simulink model "foc_sensorless_am13x"  (R2025b)
settings: Solver=FixedStepAuto  StartTime=0.0  StopTime=10  RelTol=1e-3  EnableMultiTasking=on
PostLoadFcn:
  | foc_sensorless_am13x_data;
values from neighbouring files (symbols this model uses):
  inverter = mcb.getInverterParameters('BoostXL-DRV8305')    [foc_sensorless_am13x_data.m]
  PI_params = mcb.getPIControllerParameters(pmsm, inverter, PU_System, T_pwm, Ts, Ts_speed)    [foc_sensorless_am13x_data.m]
  pmsm = mcb.getPMSMParameters('Teknic2310P')    [foc_sensorless_am13x_data.m]
  PU_System = mcb.getPUSystemParameters(pmsm, inverter)    [foc_sensorless_am13x_data.m]
  RAMP_STEP_SIZE = Id_init_assumed / N_ramp_steps    (= 0.00025)    [foc_sensorless_am13x_data.m]
  Speed_openLoop_RPM = Speed_openLoop_PU*pmsm.N_base    [foc_sensorless_am13x_data.m]
  T_pwm = 1 / PWM_frequency    (= 5e-05)    [foc_sensorless_am13x_data.m]
  Tclosedloop_stepTime = 5    [foc_sensorless_am13x_data.m]
  Ts = T_pwm    (= 5e-05)    [foc_sensorless_am13x_data.m]
  Ts_motor = T_pwm / 2    (= 2.5e-05)    [foc_sensorless_am13x_data.m]
  Ts_speed = 10 * Ts    (= 0.0005)    [foc_sensorless_am13x_data.m]
  Tspeedchange_stepTime = 7    [foc_sensorless_am13x_data.m]
undefined symbols (not defined in the file or in its folder): ADC_0_INST, DL_ADC_clearInterruptStatus, DL_ADC_INT_NUMBER1, DL_MCPWM_disableTBCLK, target
libraries: mcbcontrolslib x11, mcbeeMathTransformLib x5, simulink x5, slpidlib x3, peripheral_library_blocks_am13x x2, mcbhdlcontrolslib x2, mcbsensorlessestimatorlib x2, mcbpositiondecoderlib x2, mcbplantlib x1, autolibpmsmexterior x1, simulink_extras x1
(part 1 of 2)
settings Model: Creator=a1255762  LastModifiedBy=a1255762
settings SolverCC: AutoInsertRateTranBlk=on
settings OptimizationCC: DefaultParameterBehavior=Inlined  GainParamInheritBuiltInType=on  UseFloatMulNetSlope=on  DefaultUnderspecifiedDataType=single  UseSpecifiedMinMax=on  InlineInvariantSignals=on  StrengthReduction=on  PassReuseOutputArgsAs=Individual arguments  ZeroExternalMemoryAtStartup=off  ZeroInternalMemoryAtStartup=off  NoFixptDivByZeroProtection=on  EfficientFloat2IntCast=on  MaxStackSize=64  OptimizeBlockOrder=speed  OptimizationPriority=Speed  OptimizationCustomize=off  MultiThreadedLoops=on  AutoScheduleForLoops=on  EfficientTunableParamExpr=on
settings DebuggingCC: MultiTaskDSMMsg=none  ParameterPrecisionLossMsg=none  ParameterTunabilityLossMsg=error
settings HardwareCC: ProdBitPerPointer=32.0  ProdBitPerSizeT=32.0  ProdBitPerPtrDiffT=32.0  ProdLargestAtomicInteger=Long  ProdLargestAtomicFloat=Double  ProdWordSize=32.0  ProdLongLongMode=on  ProdHWDeviceType=ARM Compatible->ARM Cortex
settings ModelReferenceCC: ModelReferenceNumInstancesAllowed=Single
settings SFSimCC: MATLABDynamicMemAlloc=off
settings RTWCC: SystemTargetFile=ert.tlc  HardwareBoard=AM13E230x  TemplateMakefile=ert_default_tmf  Toolchain=TI ARM Clang Compiler AM13x | gmake  BuildConfiguration=Faster Runs  Description=Embedded Coder
settings CodeAppCC: ForceParamTrailComments=on  IgnoreCustomStorageClasses=off  MaxIdLength=256.0  OperatorAnnotations=on  SimulinkDataObjDesc=on  SFDataObjDesc=on  InsertBlockDesc=on
settings ERTTargetCC: ExtModeTransport=3.0  ExtModeStaticAlloc=on  ExtModeMexFile=ext_xcp  ExtModeIntrfLevel=Level2 - Open  ERTCustomFileTemplate=AM13x_codertarget_file_process.tlc  CodeReplacementLibrary=AM13x_TMU  CombineSignalStateStructs=on  SuppressErrorStatus=on  SupportAbsoluteTime=off  SubcomponentCodeInterfacePackaging=Nonreusable function  SupportNonFinite=off  SupportComplex=off

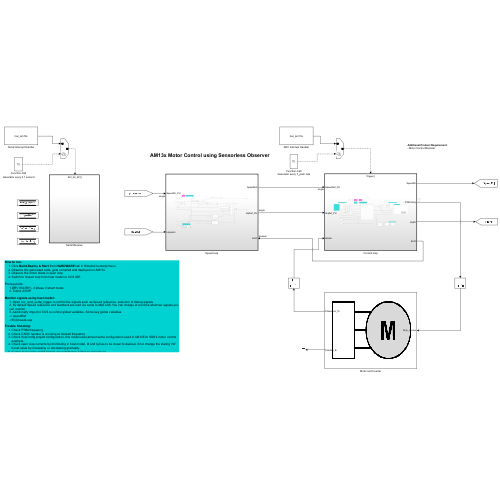
[thumbnail: Simulink's stored preview of the top-level diagram]
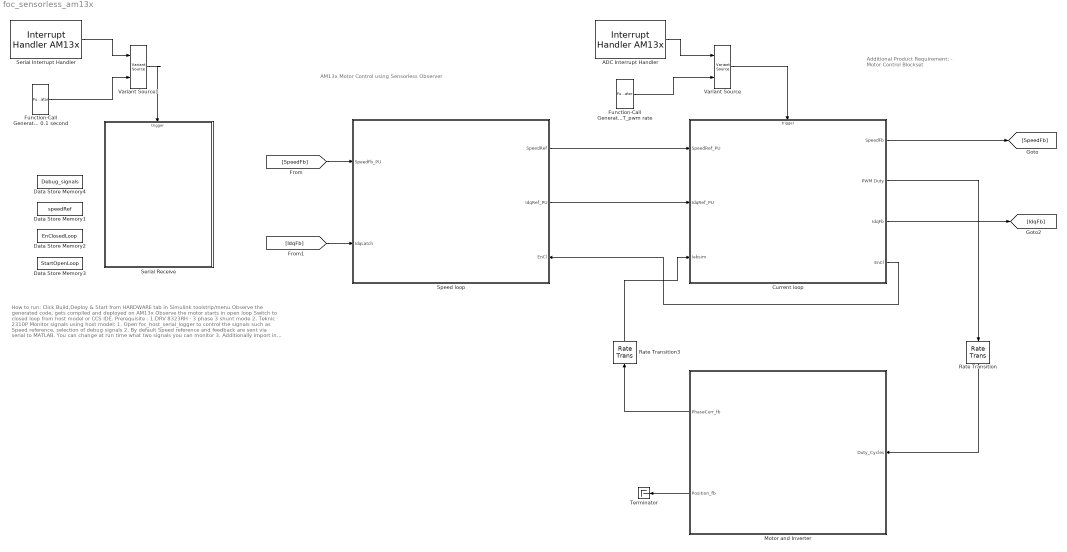
== system foc_sensorless_am13x ==
  note: Additional Product Requirement:
      | - Motor Control Blockset
  note: AM13x Motor Control using Sensorless Observer
  note: How to run:
      | Click Build,Deploy & Start from HARDWARE tab in Simulink toolstrip/menu
      | Observe the generated code, gets compiled and deployed on AM13x
      | Observe the motor starts in open loop
      | Switch to closed loop from host model or CCS IDE.
      |
      | Prerequisite :
      | 1.DRV 8323RH - 3 phase 3 shunt mode
      | 2. Teknic 2310P
      |
      | Monitor signals using host model:
      | 1. Open foc_host_serial_logger to control the signals such as Speed reference, selection of debug signals
      | 2. By default Speed reference and feedback are sent via serial to MATLAB. You can change at run time what two signals you can monitor
      | 3. Additionally import in CCS to control global variables. Some key global variables
      | -> speedRef
      | ->EnClosedLoop
      |
      | Trouble Shooting:
      | Check PWM frequency
      | Check if ADC handler is occuring at desired frequency
      | Check SysConfig project configuration, this model uses almost same configuration used in AM13E2x SDK's motor control example.
      | Check open loop currents by monitoring in host model. Id and Iq has to be closer to desired, if not change the staring Vd/boost value by increasing or decreasing gradually.
      | If open loop works and if signals are satisfactory switch to closed loop
  ADC Interrupt Handler : peripheral_library_blocks_am13x/Interrupt Handler AM13x  InterruptHandler=MTR1_FOC_INT1_Handler  PrologHandler=DL_ADC_clearInterruptStatus(ADC_0_INST, DL_ADC_INT_NUMBER1)
      settings: SourceProductName=Embedded Coder Support Package for AM13X - Peripheral Blocks
  Current loop : Subsystem
  Data Store Memory1 : DataStoreMemory  DataStoreName=speedRef  InitialValue=0.2*pmsm.N_base  ShowAdditionalParam=off  OutDataTypeStr=single
  Data Store Memory2 : DataStoreMemory  DataStoreName=EnClosedLoop  ShowAdditionalParam=off  OutDataTypeStr=boolean
  Data Store Memory3 : DataStoreMemory  DataStoreName=StartOpenLoop  ShowAdditionalParam=off  OutDataTypeStr=boolean
  Data Store Memory4 : DataStoreMemory  DataStoreName=Debug_signals  InitialValue=1  ShowAdditionalParam=off  OutDataTypeStr=uint16
  Function-Call Generator every 0.1 second : FunctionCallGenerator  SampleTime=.1
  Function-Call Generator every T_pwm rate : FunctionCallGenerator  SampleTime=T_pwm
  Motor and Inverter : Subsystem
      mask Display: image('mcb_pmsmfoc_motor.png');
  Rate Transition : RateTransition  Deterministic=off  OutPortSampleTime=Ts/2
  Rate Transition3 : RateTransition  Deterministic=off
  Serial Interrupt Handler : peripheral_library_blocks_am13x/Interrupt Handler AM13x  InterruptHandler=MW_SERIAL_RX_UC_IRQ_HANDLER  PrologHandler=Uart_Hal_InterruptHandler(&mw_am13x_serial_UartInstance)
      settings: SourceProductName=Embedded Coder Support Package for AM13X - Peripheral Blocks
  Serial Receive : Subsystem  SystemSampleTime=1e-3
  Speed loop : Subsystem  TreatAsAtomicUnit=on  SystemSampleTime=Ts_speed
      settings: PortSchema="{\"entries\":[{\"content\":{\"sides\":[{\"content\":{\"connectorIds\":[\"In1\",\"In2\"]},\"type\":\"ConnectorPlacement.EquallySpacedRectSide\",\"uuid\":\"b506ce2e-5969-464b-b6d0-26d5d9421673\"},{\"content\":{\"connectorIds\":[\"Out1\",\"Out2\",\"In3\"],\"side\":\"RIGHT\"},\"type\":\"ConnectorPlacement.EquallySpacedRectSide\",\"uuid\":\"4d96be12-936e-4168-b358-ef77535e2717\"},{\"content\":{\"side\":\"TOP\"},\"type\":\"ConnectorPlacement.EquallySpacedRectSide\",\"uuid\":\"e3c638c2-3aa9-4a35-855d-e235e847103f\"}]},\"type\":\"ConnectorPlacement.EquallySpacedConnector\",\"uuid\":\"420ee1be-7685-485e-b81d-67f311436300\"}],\"packageUris\":[\"http://schema.mathworks.com/mf0/Connector/R2020b\"],\"version\":\"1.0\"}"
  Terminator : Terminator
  Variant Source : VariantSource  VariantControlMode=sim codegen switching  OutputFunctionCall=on  VariantControls={(codegen), (sim)}
  Variant Source1 : VariantSource  VariantControlMode=sim codegen switching  OutputFunctionCall=on  VariantControls={(codegen), (sim)}
  wires:
  Rate Transition/1 -> Motor and Inverter/1(Duty_Cycles)
  Current loop/1(SpeedFb) -> [SpeedFb]
  Current loop/2(PWM Duty) -> Rate Transition/1
  Current loop/3(IdqFb) -> [IdqFb]
  ADC Interrupt Handler/1 -> Variant Source/1
  Function-Call Generator every T_pwm rate/1 -> Variant Source/2
  Variant Source/1 -> Current loop/Trigger
  Motor and Inverter/1(PhaseCurr_fb) -> Rate Transition3/1
  Rate Transition3/1 -> Current loop/3(Iabsim)
  [SpeedFb] -> Speed loop/1(SpeedFb_PU)
  [IdqFb] -> Speed loop/2(IdqLatch)
  Motor and Inverter/2(Position_fb) -> Terminator/1
  Speed loop/1(SpeedRef) -> Current loop/1(SpeedRef_PU)
  Speed loop/2(IdqRef_PU) -> Current loop/2(IdqRef_PU)
  Current loop/4(EnCl) -> Speed loop/3(EnCl)
  Function-Call Generator every 0.1 second/1 -> Variant Source1/2
  Serial Interrupt Handler/1 -> Variant Source1/1
  Variant Source1/1 -> Serial Receive/Trigger

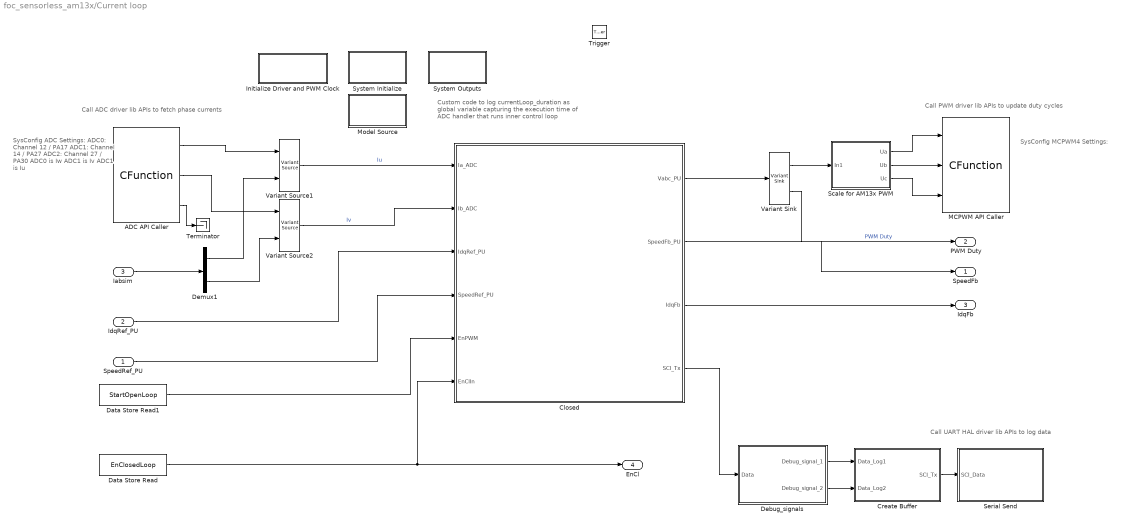
== system foc_sensorless_am13x/Current loop ==
  note: SysConfig ADC Settings:
      |
      | ADC0: Channel 12 / PA17
      | ADC1: Channel 14 / PA27
      | ADC2: Channel 27 / PA30
      |
      |
      | ADC0 is Iw
      | ADC1 is Iv
      | ADC1 is Iu
  note: Custom code to log currentLoop_duration as global variable capturing the execution time of ADC handler that runs inner control loop
  note: Call ADC driver lib APIs to fetch phase currents
  note: Call PWM driver lib APIs to update duty cycles
  note: Call UART HAL driver lib APIs to log data
  note: SysConfig MCPWM4 Settings:
  SpeedRef_PU : Inport  OutDataTypeStr=single
  IdqRef_PU : Inport  Port=2
  Iabsim : Inport  Port=3
  Trigger : TriggerPort  TriggerType=function-call  VariantControl=(inherit)  PortDimensions=1
  " ADC API Caller" : CFunction  CodeGenUsesSimCustomCode=off  CodegenOutputCode=|  CustomHeaderFile=|
      CodegenOutputCode=|
      | /* Read ADC conversion results from respective result registers */ 
      | Iw = DL_ADC_readResult(ADC_0_RESULT_INST, DL_ADC_SOC_NUMBER0);
      | Iv = DL_ADC_readResult(ADC_1_RESULT_INST, DL_ADC_SOC_NUMBER0);
      | Iu = DL_ADC_readResult(ADC_2_RESULT_INST, DL_ADC_SOC_NUMBER0);
      CustomHeaderFile=|
      | dl_adc.h
      | hw_memmap.h
      | ti_sdk_dl_config.h
  "Closed " : Subsystem  RTWFcnName=MTR1_FOC_INT1_Handler
      settings: RTWFcnNameOpts=User specified
  Create Buffer : Subsystem
  Data Store Read : DataStoreRead  DataStoreName=EnClosedLoop  IndexOptions=Index vector (dialog)  Indices=1  OutputSizes=1
  Data Store Read1 : DataStoreRead  DataStoreName=StartOpenLoop  IndexOptions=Index vector (dialog)  Indices=1  OutputSizes=1
  Debug_signals : Subsystem
  Demux1 : Demux  Outputs=2
  Initialize Driver and PWM Clock : Subsystem  TreatAsAtomicUnit=on
  MCPWM API Caller : CFunction  CodeGenUsesSimCustomCode=off  CodegenOutputCode=|  CustomHeaderFile=|
      CodegenOutputCode=|
      | DL_MCPWM_setCounterCompareShadowValue(MTR1_MCPWM_BASE_INST, DL_MCPWM_COUNTER_COMPARE_1A, Ua);
      | DL_MCPWM_setCounterCompareShadowValue(MTR1_MCPWM_BASE_INST, DL_MCPWM_COUNTER_COMPARE_1B, Ua);
      | DL_MCPWM_setCounterCompareShadowValue(MTR1_MCPWM_BASE_INST, DL_MCPWM_COUNTER_COMPARE_2A, Ub);
      | DL_MCPWM_setCounterCompareShadowValue(MTR1_MCPWM_BASE_INST, DL_MCPWM_COUNTER_COMPARE_2B, Ub);
      | DL_MCPWM_setCounterCompareShadowValue(MTR1_MCPWM_BASE_INST, DL_MCPWM_COUNTER_COMPARE_3A, Uc);
      | DL_MCPWM_setCounterCompareShadowValue(MTR1_MCPWM_BASE_INST, DL_MCPWM_COUNTER_COMPARE_3B, Uc);
      CustomHeaderFile=|
      | dl_mcpwm.h
      | hw_memmap.h
      | ti_sdk_dl_config.h
  Model Source : Subsystem  mask(Model Source){ShowInLibBrowser=0}
      mask prompts: ShowInLibBrowser "Simulink:masks:CustCodeMaskParam1_MP"
      settings: CopyFcn=cccopyfcn(gcb)  OpenFcn=ccopenfcn('Model Source')
      mask Help: eval('feval(''rtwprivate'',''rtwhelpview'',''rtw_model_source_block'')');
      mask Display: disp('Model\nSource');
  Scale for AM13x PWM : Subsystem
  Serial Send : Subsystem
  System Initialize : Subsystem  mask(System Initialize){ShowInLibBrowser=0}
      mask prompts: ShowInLibBrowser "Simulink:masks:CustCodeMaskParam1_MP"
      settings: CopyFcn=cccopyfcn(gcb)  OpenFcn=ccopenfcn('System Initialize Function')
      mask Help: eval('feval(''rtwprivate'',''rtwhelpview'',''rtw_sys_initialize_block'')');
      mask Display: disp('System\nInitialize');
  System Outputs : Subsystem  mask(System Outputs){ShowInLibBrowser=0}
      mask prompts: ShowInLibBrowser "Simulink:masks:CustCodeMaskParam1_MP"
      settings: CopyFcn=cccopyfcn(gcb)  OpenFcn=ccopenfcn('System Outputs Function')
      mask Help: eval('feval(''rtwprivate'',''rtwhelpview'',''rtw_sys_outputs_block'')');
      mask Display: disp('System\nOutputs');
  Terminator : Terminator
  Variant Sink : VariantSink  VariantControlMode=sim codegen switching  VariantControls={(codegen), (sim)}
  Variant Source1 : VariantSource  VariantControlMode=sim codegen switching  VariantControls={(codegen), (sim)}
  Variant Source2 : VariantSource  VariantControlMode=sim codegen switching  VariantControls={(codegen), (sim)}
  SpeedFb : Outport
  PWM Duty : Outport  Port=2
  IdqFb : Outport  Port=3
  EnCl : Outport  Port=4
  wires:
  " ADC API Caller"/1 -> Variant Source1/1
  Demux1/1 -> Variant Source1/2
  Variant Sink/2 -> PWM Duty/1  "PWM Duty"
  " ADC API Caller"/2 -> Variant Source2/1
  Variant Source1/1 -> "Closed "/1(Ia_ADC)  "Iu"
  Variant Source2/1 -> "Closed "/2(Ib_ADC)  "Iv"
  "Closed "/1(Vabc_PU) -> Variant Sink/1
  "Closed "/2(SpeedFb_PU) -> SpeedFb/1
  "Closed "/3(IdqFb) -> IdqFb/1
  IdqRef_PU/1 -> "Closed "/3(IdqRef_PU)
  SpeedRef_PU/1 -> "Closed "/4(SpeedRef_PU)
  Data Store Read/1 -> EnCl/1, "Closed "/6(EnClIn)
  Demux1/2 -> Variant Source2/2
  Iabsim/1 -> Demux1/1
  Create Buffer/1(SCI_Tx) -> Serial Send/1(SCI_Data)
  "Closed "/4(SCI_Tx) -> Debug_signals/1(Data)
  Debug_signals/2(Debug_signal_2) -> Create Buffer/2(Data_Log2)
  Debug_signals/1(Debug_signal_1) -> Create Buffer/1(Data_Log1)
  " ADC API Caller"/3 -> Terminator/1
  Variant Sink/1 -> Scale for AM13x PWM/1(In1)
  Scale for AM13x PWM/1(Ua) -> MCPWM API Caller/1
  Scale for AM13x PWM/2(Ub) -> MCPWM API Caller/2
  Scale for AM13x PWM/3(Uc) -> MCPWM API Caller/3
  Data Store Read1/1 -> "Closed "/5(EnPWM)

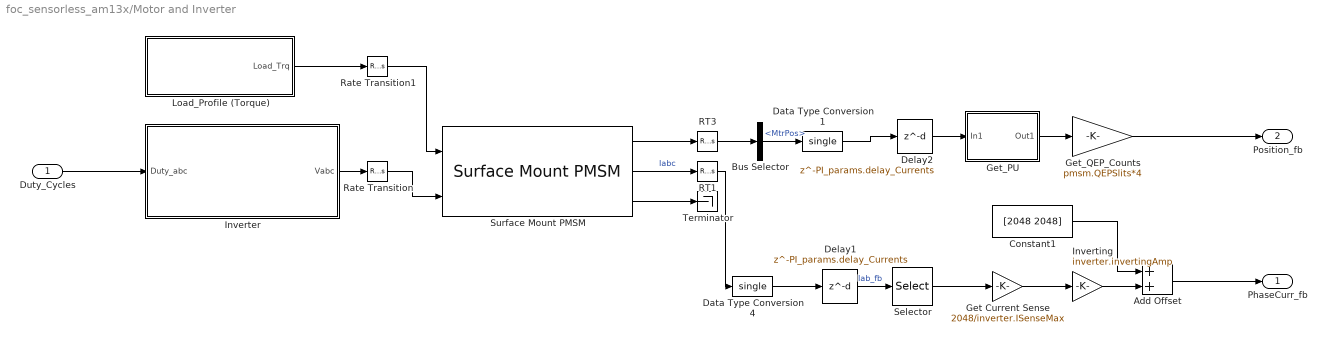
== system foc_sensorless_am13x/Motor and Inverter ==
  Duty_Cycles : Inport
  Add Offset : Sum  OutDataTypeStr=Inherit: Same as first input
  Bus Selector : BusSelector  OutputSignals=MtrPos
  Constant1 : Constant  Value=[2048 2048]  OutDataTypeStr=uint16
  Data Type Conversion1 : DataTypeConversion  OutDataTypeStr=single  RndMeth=Simplest  SaturateOnIntegerOverflow=off
  Data Type Conversion4 : DataTypeConversion  OutDataTypeStr=single  RndMeth=Simplest  SaturateOnIntegerOverflow=off
  Delay1 : Delay  DelayLength=PI_params.delay_Currents
  Delay2 : Delay  DelayLength=PI_params.delay_Currents
  "Get Current Sense " : Gain  Gain=2048/inverter.ISenseMax  OutDataTypeStr=int16  RndMeth=Simplest
  Get_PU : Subsystem
  Get_QEP_Counts : Gain  Gain=pmsm.QEPSlits*4  OutDataTypeStr=uint16  RndMeth=Simplest
  Inverter : Subsystem
  Inverting : Gain  Gain=inverter.invertingAmp  OutDataTypeStr=int16  RndMeth=Simplest
  Load_Profile (Torque) : Subsystem
  RT1 : RateTransition  Deterministic=off  OutPortSampleTime=Ts_motor
  RT3 : RateTransition  Deterministic=off  OutPortSampleTime=Ts_motor
  Rate Transition : RateTransition  Deterministic=off  OutPortSampleTime=Ts_motor
  Rate Transition1 : RateTransition  Deterministic=off  OutPortSampleTime=Ts_motor
  Selector : Selector  InputPortWidth=3  IndexOptions=Index vector (dialog)  Indices=[1 2]  OutputSizes=1
  Surface Mount PMSM : autolibpmsmexterior/Surface Mount PMSM  port_config=Torque  sim_type=Discrete  Ts=Ts_motor  P=pmsm.p  Rs=pmsm.Rs  Ldq_=pmsm.Ld  KConstText=Back-emf constant (Ke):  lambda_pm=pmsm.FluxPM  Ke=pmsm.Ke  Kt=1.323  mechanical=[pmsm.J, pmsm.B, 0]  idq0=[0 0]  theta_init=0  omega_init=0  KConst=pmsm.FluxPM  lambda_pm_calc=0.0096483  RefBlkName='autolibpmsmexterior/Surface Mount PMSM'  aMode=5  Ldq="[0.0002      0.0002]"
  Terminator : Terminator
  PhaseCurr_fb : Outport
  Position_fb : Outport  Port=2
  wires:
  Data Type Conversion1/1 -> Delay2/1
  Bus Selector/1 -> Data Type Conversion1/1  "<MtrPos>"
  Delay1/1 -> Selector/1  "Iab_fb"
  Data Type Conversion4/1 -> Delay1/1
  Duty_Cycles/1 -> Inverter/1(Duty_abc)
  RT3/1 -> Bus Selector/1
  Rate Transition1/1 -> Surface Mount PMSM/1
  Surface Mount PMSM/3 -> Terminator/1
  Surface Mount PMSM/2 -> RT1/1  "Iabc"
  Inverter/1(Vabc) -> Rate Transition/1
  Load_Profile (Torque)/1(Load_Trq) -> Rate Transition1/1
  Rate Transition/1 -> Surface Mount PMSM/2
  Surface Mount PMSM/1 -> RT3/1
  RT1/1 -> Data Type Conversion4/1
  Get_QEP_Counts/1 -> Position_fb/1
  "Get Current Sense "/1 -> Inverting/1
  Constant1/1 -> Add Offset/1
  Delay2/1 -> Get_PU/1(In1)
  Get_PU/1(Out1) -> Get_QEP_Counts/1
  Add Offset/1 -> PhaseCurr_fb/1
  Selector/1 -> "Get Current Sense "/1
  Inverting/1 -> Add Offset/2

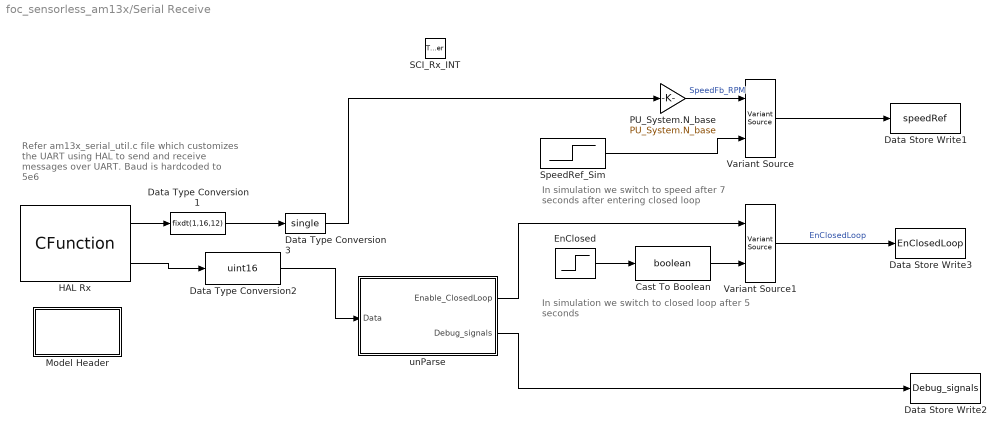
== system foc_sensorless_am13x/Serial Receive ==
  note: Refer am13x_serial_util.c file which customizes the UART using HAL to send and receive messages over UART. Baud is hardcoded to 5e6
  note: In simulation we switch to speed after 7 seconds after entering closed loop
  note: In simulation we switch to closed loop after 5 seconds
  SCI_Rx_INT : TriggerPort  TriggerType=function-call  VariantControl=Variant
  Cast To Boolean : DataTypeConversion  OutDataTypeStr=boolean  SaturateOnIntegerOverflow=off  RndMeth=Floor
  Data Store Write1 : DataStoreWrite  DataStoreName=speedRef  IndexOptions=Index vector (dialog)  Indices=1  OutputSizes=1
  Data Store Write2 : DataStoreWrite  DataStoreName=Debug_signals  IndexOptions=Index vector (dialog)  Indices=1  OutputSizes=1
  Data Store Write3 : DataStoreWrite  DataStoreName=EnClosedLoop  IndexOptions=Index vector (dialog)  Indices=1  OutputSizes=1
  Data Type Conversion1 : DataTypeConversion  OutDataTypeStr=fixdt(1,16,12)  ConvertRealWorld=Stored Integer (SI)  RndMeth=Simplest  SaturateOnIntegerOverflow=off
  Data Type Conversion2 : DataTypeConversion  OutDataTypeStr=uint16  RndMeth=Simplest  SaturateOnIntegerOverflow=off
  Data Type Conversion3 : DataTypeConversion  OutDataTypeStr=single  RndMeth=Simplest  SaturateOnIntegerOverflow=off
  EnClosed : Step  Time=Tclosedloop_stepTime  OutDataTypeStr=single
  HAL Rx : CFunction  CodeGenUsesSimCustomCode=off  CodegenOutputCode=mw_am13x_serial_GetRxData(&SCI_Rx1, &SCI_Rx2);  CustomHeaderFile=|
      | hw_memmap.h
      | ti_sdk_dl_config.h
      | Uart_Hal.h
  Model Header : Subsystem  mask(Model Header){ShowInLibBrowser=0}
      mask prompts: ShowInLibBrowser "Simulink:masks:CustCodeMaskParam1_MP"
      settings: CopyFcn=cccopyfcn(gcb)  OpenFcn=ccopenfcn('Model Header')
      mask Help: eval('feval(''rtwprivate'',''rtwhelpview'',''rtw_model_header_block'')');
      mask Display: disp('Model\nHeader');
  PU_System.N_base : Gain  Gain=PU_System.N_base
  SpeedRef_Sim : Step  Time=Tspeedchange_stepTime  Before=0.2*pmsm.N_base  After=0.3*pmsm.N_base  OutDataTypeStr=single
  Variant Source : VariantSource  VariantControlMode=sim codegen switching  VariantControls={(codegen), (sim)}
  Variant Source1 : VariantSource  VariantControlMode=sim codegen switching  VariantControls={(codegen), (sim)}
  unParse : Subsystem
  wires:
  Data Type Conversion3/1 -> PU_System.N_base/1
  HAL Rx/1 -> Data Type Conversion1/1
  unParse/2(Debug_signals) -> Data Store Write2/1
  Data Type Conversion2/1 -> unParse/1(Data)
  Data Type Conversion1/1 -> Data Type Conversion3/1
  HAL Rx/2 -> Data Type Conversion2/1
  SpeedRef_Sim/1 -> Variant Source/2
  Variant Source/1 -> Data Store Write1/1
  PU_System.N_base/1 -> Variant Source/1  "SpeedFb_RPM"
  Variant Source1/1 -> Data Store Write3/1  "EnClosedLoop"
  EnClosed/1 -> Cast To Boolean/1
  unParse/1(Enable_ClosedLoop) -> Variant Source1/1
  Cast To Boolean/1 -> Variant Source1/2

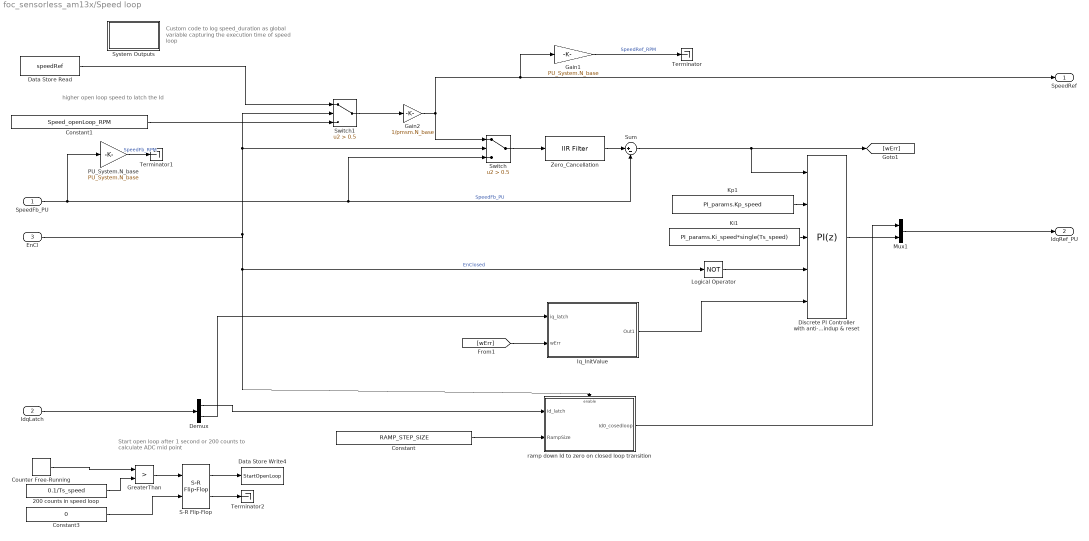
== system foc_sensorless_am13x/Speed loop ==
  note: higher open loop speed to latch the Id
  note: Start open loop after 1 second or 200 counts to calculate ADC mid point
  note: Custom code to log speed_duration as global variable capturing the execution time of speed loop
  SpeedFb_PU : Inport  OutDataTypeStr=single
  IdqLatch : Inport  Port=2
  EnCl : Inport  Port=3  OutDataTypeStr=boolean
  200 counts in speed loop : Constant  Value=0.1/Ts_speed  OutDataTypeStr=uint16
  Constant : Constant  Value=RAMP_STEP_SIZE  OutDataTypeStr=single
  Constant1 : Constant  Value=Speed_openLoop_RPM  OutDataTypeStr=single
  Constant3 : Constant  Value=0  OutDataTypeStr=boolean
  Counter Free-Running : simulink/Sources/Counter Free-Running  NumBits=16  tsamp=-1
  Data Store Read : DataStoreRead  DataStoreName=speedRef  IndexOptions=Index vector (dialog)  Indices=1  OutputSizes=1
  Data Store Write4 : DataStoreWrite  DataStoreName=StartOpenLoop  IndexOptions=Index vector (dialog)  Indices=1  OutputSizes=1
  Demux : Demux  Outputs=2
  Discrete PI Controller with anti-windup & reset : slpidlib/PID Controller  Controller=PI  Form=Parallel  TimeDomain=Discrete-time  UseExternalTs=off  SampleTime=-1  IntegratorMethod=Forward Euler  FilterMethod=Forward Euler  ControllerParametersSource=external  P=1  I=1  UseKiTs=on  D=0  UseExternalDerivativeSource=off  N=100  UseFilter=on  TunerSelectOption=Transfer Function Based (PID Tuner App)  InitialConditionSource=external  InitialConditionForIntegrator=0  InitialConditionForFilter=0  DifferentiatorICPrevScaledInput=0  ExternalReset=level  TrackingMode=off  Kt=1  LimitOutput=on  SatLimitsSource=internal  UpperSaturationLimit=pmsm.I_rated/inverter.ISenseMax  LowerSaturationLimit=-pmsm.I_rated/inverter.ISenseMax  LinearizeAsGain=on  AntiWindupMode=clamping  Kb=1  LimitIntegrator=off  UpperIntegratorSaturationLimit=inf  LowerIntegratorSaturationLimit=-inf  RndMeth=Simplest  POutMin=[]  POutMax=[]  IOutMin=[]  IOutMax=[]  DOutMin=[]  DOutMax=[]  NOutMin=[]  NOutMax=[]  SumOutMin=[]  SumOutMax=[]  SaturationOutDataTypeStr=Inherit: Inherit via back propagation  SaturationOutMin=[]  SaturationOutMax=[]  PParamMin=[]  PParamMax=[]  IParamMin=[]  IParamMax=[]  DParamMin=[]  DParamMax=[]  NParamMin=[]  NParamMax=[]  KbParamMin=[]  KbParamMax=[]  KtParamMin=[]  KtParamMax=[]  KbOutMin=[]  KbOutMax=[]  KtOutMin=[]  KtOutMax=[]  IntegratorOutMin=[]  IntegratorOutMax=[]  FilterOutMin=[]  FilterOutMax=[]  SumI1OutMin=[]  SumI1OutMax=[]  SumI2OutMin=[]  SumI2OutMax=[]  SumI3OutMin=[]  SumI3OutMax=[]  SumI4OutMin=[]  SumI4OutMax=[]  SumDOutMin=[]  SumDOutMax=[]  DifferentiatorOutMin=[]  DifferentiatorOutMax=[]  FilterDiffOutCoefMin=[]  FilterDiffOutCoefMax=[]  ReciprocalOutMin=[]  ReciprocalOutMax=[]  SumDenOutMin=[]  SumDenOutMax=[]  SumNumOutMin=[]  SumNumOutMax=[]  DivideOutMin=[]  DivideOutMax=[]  UdiffTsProdOutMin=[]  UdiffTsProdOutMax=[]  NTsProdOutMin=[]  NTsProdOutMax=[]  UintegralTsProdOutMin=[]  UintegralTsProdOutMax=[]  UngainTsProdOutMin=[]  UngainTsProdOutMax=[]  ClampingZeroOutDataTypeStr=Inherit: Inherit via back propagation  ClampingZeroOutMin=[]  ClampingZeroOutMax=[]  FilterDenConstantOutDataTypeStr=Inherit: Inherit via back propagation  FilterDenConstantOutMin=[]  FilterDenConstantOutMax=[]  PCopyOutDataTypeStr=Inherit: Inherit via back propagation  PCopyOutMin=[]  PCopyOutMax=[]  NCopyOutDataTypeStr=Inherit: Inherit via back propagation  NCopyOutMin=[]  NCopyOutMax=[]  IntegratorContinuousStateAttributes=''  IntegratorStateMustResolveToSignalObject=off  IntegratorRTWStateStorageClass=Auto  FilterContinuousStateAttributes=''  FilterStateMustResolveToSignalObject=off  FilterRTWStateStorageClass=Auto  ParallelPVariant=ExternalParameters  IdealPVariant=Disabled  IVariant=ExternalParameters  DVariant=Disabled  IntegratorVariant=Discrete  SatVariant=Enabled  AWVariant=DiscClampingParallel  PCopyVariant=Disabled  TRVariant=Disabled  FdbkBlocksVariant=Forward  IdealPFdbkVariant=Disabled  SatFdbkVariant=Disabled  DerivativeFilterVariant=Disabled  NVariant=Disabled  NCopyVariant=Disabled_SignalSpec  FilterICVariant=Disabled  IntegratorICVariant=ExternalICs  ExternalResetVariant=ExternalReset  TRSumVariant=Passthrough  SumFdbkVariant=Disabled  SumVariant=Sum_PI  TsampFilterVariant=InternalTs  TsampNgainVariant=Passthrough  TsampIntegralVariant=Disabled_SignalSpec  ExternalSaturationOutDataTypeStr=Inherit: Same as second input  DerivativeSourceVariant=Disabled  PreIntVariant=InternalPreInt
      settings: LibrarySourceBlock=mcbcontrolslib/PI Controller
  Gain1 : Gain  Gain=PU_System.N_base
  Gain2 : Gain  Gain=1/pmsm.N_base
  GreaterThan : RelationalOperator  Operator=>  OutDataTypeStr=boolean  RndMeth=Simplest  InputSameDT=off
  Iq_InitValue : Subsystem
  Ki1 : Constant  Value=PI_params.Ki_speed*single(Ts_speed)  OutDataTypeStr=dataType  SampleTime=-1
  Kp1 : Constant  Value=PI_params.Kp_speed  OutDataTypeStr=dataType  SampleTime=-1
  Logical Operator : Logic  Operator=NOT  IconShape=distinctive  AllPortsSameDT=off  OutDataTypeStr=boolean
  Mux1 : Mux  Inputs=2
  PU_System.N_base : Gain  Gain=PU_System.N_base
  S-R Flip-Flop : simulink_extras/Flip Flops/S-R Flip-Flop  initial_condition=0
  Sum : Sum  Inputs=|+-  OutDataTypeStr=Inherit: Same as first input
  Switch : Switch  Criteria=u2 > Threshold  Threshold=0.5  SaturateOnIntegerOverflow=off  InputSameDT=off
  Switch1 : Switch  Criteria=u2 > Threshold  Threshold=0.5  SaturateOnIntegerOverflow=off  InputSameDT=off
  System Outputs : Subsystem  mask(System Outputs){ShowInLibBrowser=0}
      mask prompts: ShowInLibBrowser "Simulink:masks:CustCodeMaskParam1_MP"
      settings: CopyFcn=cccopyfcn(gcb)  OpenFcn=ccopenfcn('System Outputs Function')
      mask Help: eval('feval(''rtwprivate'',''rtwhelpview'',''rtw_sys_outputs_block'')');
      mask Display: disp('System\nOutputs');
  Terminator : Terminator
  Terminator1 : Terminator
  Terminator2 : Terminator
  Zero_Cancellation : mcbcontrolslib/IIR Filter  VariantControl=Low Pass Filter  VariantSelect=Low-pass  FilterConstantInputType=Specify via dialog  Filter_constant=0.01*(Ts_speed/Ts)  InitialOutput=Specify via dialog  InitialOutputValue=0  ExternalReset=none  advancedSettings=off  Ts=50e-6  cutOff_freq=353.6777
  ramp down Id to zero on closed loop transition : Subsystem
  SpeedRef : Outport
  IdqRef_PU : Outport  Port=2  OutDataTypeStr=single  VectorParamsAs1DForOutWhenUnconnected=off
  wires:
  Mux1/1 -> IdqRef_PU/1
  Kp1/1 -> Discrete PI Controller with anti-windup & reset/2
  PU_System.N_base/1 -> Terminator1/1  "SpeedFb_RPM"
  Logical Operator/1 -> Discrete PI Controller with anti-windup & reset/4
  Gain1/1 -> Terminator/1  "SpeedRef_RPM"
  SpeedFb_PU/1 -> PU_System.N_base/1, Sum/2, Switch/3  "SpeedFb_PU"
  Discrete PI Controller with anti-windup & reset/1 -> Mux1/2
  Sum/1 -> Discrete PI Controller with anti-windup & reset/1, [wErr]
  Ki1/1 -> Discrete PI Controller with anti-windup & reset/3
  EnCl/1 -> ramp down Id to zero on closed loop transition/Enable, Logical Operator/1, Switch/2, Switch1/2  "EnClosed"
  Switch1/1 -> Gain2/1
  Gain2/1 -> Switch/1, Gain1/1, SpeedRef/1
  Switch/1 -> Zero_Cancellation/1
  IdqLatch/1 -> Demux/1
  Demux/1 -> ramp down Id to zero on closed loop transition/1(Id_latch)
  Constant/1 -> ramp down Id to zero on closed loop transition/2(RampSize)
  Constant1/1 -> Switch1/3
  Demux/2 -> Iq_InitValue/1(iq_latch)
  Iq_InitValue/1(Out1) -> Discrete PI Controller with anti-windup & reset/5
  ramp down Id to zero on closed loop transition/1(Id0_cosedloop) -> Mux1/1
  [wErr] -> Iq_InitValue/2(wErr)
  Data Store Read/1 -> Switch1/1
  Zero_Cancellation/1 -> Sum/1
  S-R Flip-Flop/1 -> Data Store Write4/1
  S-R Flip-Flop/2 -> Terminator2/1
  Counter Free-Running/1 -> GreaterThan/1
  GreaterThan/1 -> S-R Flip-Flop/1
  200 counts in speed loop/1 -> GreaterThan/2
  Constant3/1 -> S-R Flip-Flop/2

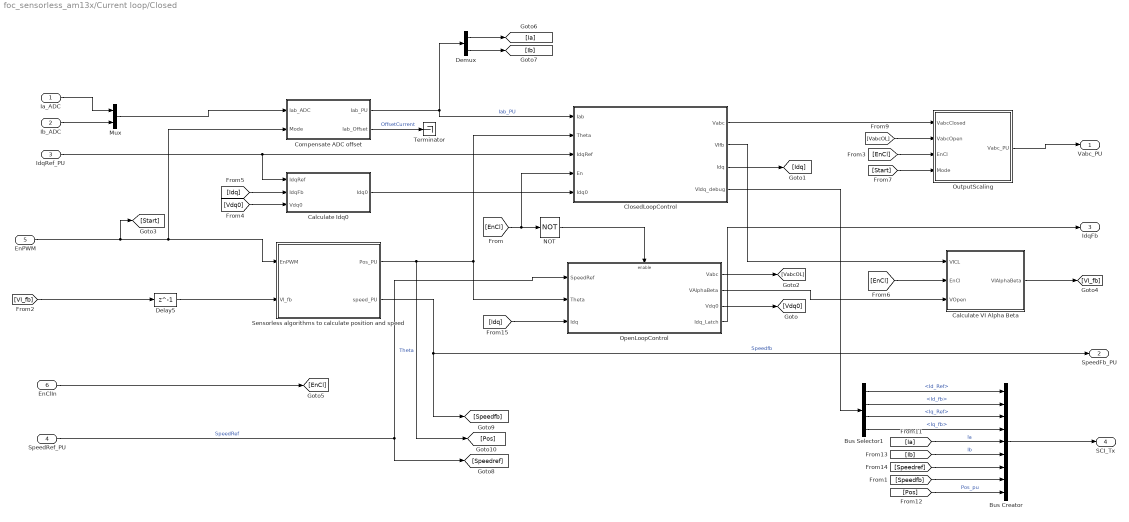
== system foc_sensorless_am13x/Current loop/Closed  ==
  Ia_ADC : Inport
  Ib_ADC : Inport  Port=2
  IdqRef_PU : Inport  Port=3  OutDataTypeStr=dataType  PortDimensions=2
  SpeedRef_PU : Inport  Port=4  OutDataTypeStr=single
  EnPWM : Inport  Port=5
  EnClIn : Inport  Port=6
  Bus Creator : BusCreator  Inputs=9
  Bus Selector1 : BusSelector  OutputSignals=Id_Ref,Id_fb,Iq_Ref,Iq_fb
  Calculate Idq0 : Subsystem
  Calculate VI Alpha Beta : Subsystem
  ClosedLoopControl : Subsystem
  Compensate ADC offset : Subsystem
  Delay5 : Delay  DelayLength=1
  Demux : Demux  Outputs=2
  Mux : Mux  Inputs=2
  NOT : Logic  Operator=NOT  IconShape=distinctive  AllPortsSameDT=off  OutDataTypeStr=boolean
  OpenLoopControl : Subsystem
  OutputScaling : Subsystem
  Sensorless algorithms to calculate position and speed : Subsystem
  Terminator : Terminator
  Vabc_PU : Outport  OutDataTypeStr=single  VectorParamsAs1DForOutWhenUnconnected=off
  SpeedFb_PU : Outport  Port=2
  IdqFb : Outport  Port=3
  SCI_Tx : Outport  Port=4
  wires:
  NOT/1 -> OpenLoopControl/Enable
  OpenLoopControl/2(VAlphaBeta) -> Calculate VI Alpha Beta/3(VOpen)
  [EnCl] -> OutputScaling/3(EnCl)
  Compensate ADC offset/1(Iab_PU) -> Demux/1, ClosedLoopControl/1(Iab)  "Iab_PU"
  [Vdq0] -> Calculate Idq0/3(Vdq0)
  Delay5/1 -> Sensorless algorithms to calculate position and speed/2(VI_fb)
  OpenLoopControl/3(Vdq0) -> [Vdq0]
  Sensorless algorithms to calculate position and speed/1(Pos_PU) -> [Pos], OpenLoopControl/2(Theta), ClosedLoopControl/2(Theta)  "Theta"
  SpeedRef_PU/1 -> [Speedref], OpenLoopControl/1(SpeedRef)  "SpeedRef"
  Calculate Idq0/1(Idq0) -> ClosedLoopControl/5(Idq0)
  [EnCl] -> Calculate VI Alpha Beta/2(EnCl)
  IdqRef_PU/1 -> ClosedLoopControl/3(IdqRef), Calculate Idq0/1(IdqRef)
  [VI_fb] -> Delay5/1
  [VabcOL] -> OutputScaling/2(VabcOpen)
  OutputScaling/1(Vabc_PU) -> Vabc_PU/1
  ClosedLoopControl/3(Idq) -> [Idq]
  [EnCl] -> ClosedLoopControl/4(En), NOT/1
  OpenLoopControl/1(Vabc) -> [VabcOL]
  [Idq] -> Calculate Idq0/2(IdqFb)
  EnClIn/1 -> [EnCl]
  Ib_ADC/1 -> Mux/2
  Ia_ADC/1 -> Mux/1
  Sensorless algorithms to calculate position and speed/2(speed_PU) -> [Speedfb], SpeedFb_PU/1  "Speedfb"
  [Speedfb] -> Bus Creator/8
  [Ia] -> Bus Creator/5  "Ia"
  [Speedref] -> Bus Creator/7
  [Ib] -> Bus Creator/6  "Ib"
  [Pos] -> Bus Creator/9  "Pos_pu"
  Bus Creator/1 -> SCI_Tx/1
  Calculate VI Alpha Beta/1(VIAlphaBeta) -> [VI_fb]
  Demux/1 -> [Ia]
  Mux/1 -> Compensate ADC offset/1(Iab_ADC)
  Demux/2 -> [Ib]
  Bus Selector1/1 -> Bus Creator/1  "<Id_Ref>"
  Bus Selector1/2 -> Bus Creator/2  "<Id_fb>"
  Bus Selector1/3 -> Bus Creator/3  "<Iq_Ref>"
  Bus Selector1/4 -> Bus Creator/4  "<Iq_fb>"
  ClosedLoopControl/1(Vabc) -> OutputScaling/1(VabcClosed)
  ClosedLoopControl/2(VIfb) -> Calculate VI Alpha Beta/1(VICL)
  ClosedLoopControl/4(VIdq_debug) -> Bus Selector1/1
  Compensate ADC offset/2(Iab_Offset) -> Terminator/1  "OffsetCurrent"
  [Idq] -> OpenLoopControl/3(Idq)
  OpenLoopControl/4(Idq_Latch) -> IdqFb/1
  [Start] -> OutputScaling/4(Mode)
  EnPWM/1 -> [Start], Compensate ADC offset/2(Mode), Sensorless algorithms to calculate position and speed/1(EnPWM)

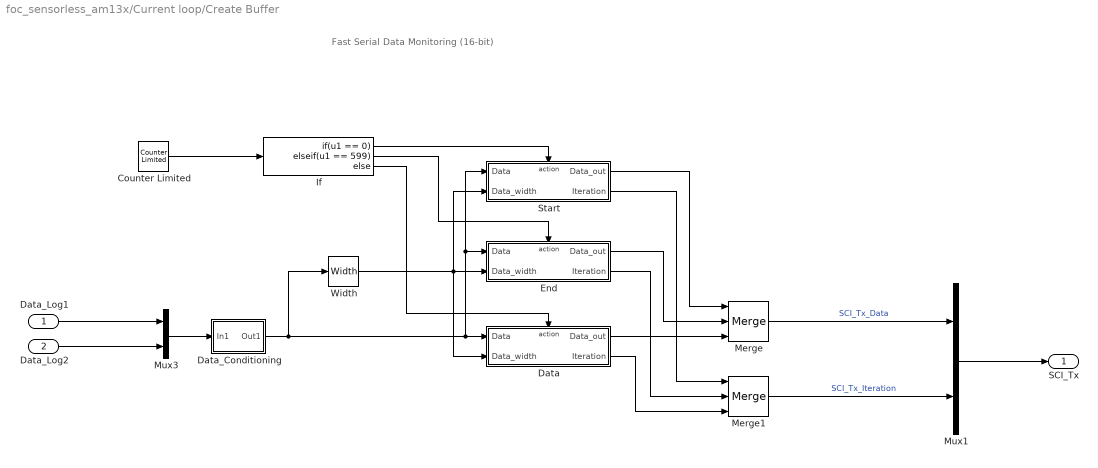
== system foc_sensorless_am13x/Current loop/Create Buffer ==
  note: Fast Serial Data Monitoring (16-bit)
  Data_Log1 : Inport
  Data_Log2 : Inport  Port=2
  Counter Limited : simulink/Sources/Counter Limited  uplimit=599  tsamp=-1
  Data : Subsystem  TreatAsAtomicUnit=on
  Data_Conditioning : Subsystem
  End : Subsystem  TreatAsAtomicUnit=on
  If : If  IfExpression=u1 == 0  ElseIfExpressions=u1 == 599
  Merge : Merge  Inputs=3
  Merge1 : Merge  Inputs=3
  Mux1 : Mux  Inputs=2
  Mux3 : Mux  Inputs=2
  Start : Subsystem  TreatAsAtomicUnit=on
  Width : Width  OutDataTypeMode=All ports same datatype  DataType=uint16
  SCI_Tx : Outport
  wires:
  Data_Conditioning/1(Out1) -> Width/1, Data/1(Data), End/1(Data), Start/1(Data)
  Counter Limited/1 -> If/1
  Data_Log1/1 -> Mux3/1
  Data/1(Data_out) -> Merge/3
  Data_Log2/1 -> Mux3/2
  Width/1 -> Data/2(Data_width), End/2(Data_width), Start/2(Data_width)
  Data/2(Iteration) -> Merge1/3
  End/2(Iteration) -> Merge1/2
  If/1 -> Start/Action
  Start/1(Data_out) -> Merge/1
  Merge1/1 -> Mux1/2  "SCI_Tx_Iteration"
  Mux3/1 -> Data_Conditioning/1(In1)
  Start/2(Iteration) -> Merge1/1
  If/2 -> End/Action
  End/1(Data_out) -> Merge/2
  If/3 -> Data/Action
  Mux1/1 -> SCI_Tx/1
  Merge/1 -> Mux1/1  "SCI_Tx_Data"

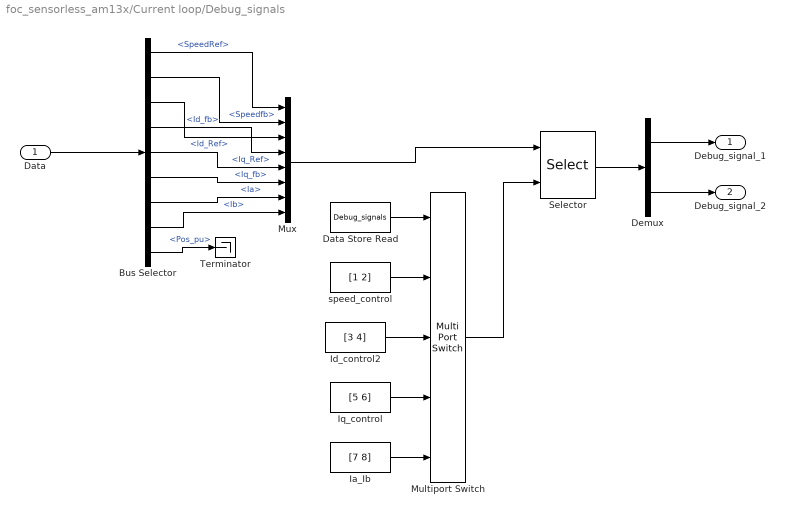
== system foc_sensorless_am13x/Current loop/Debug_signals ==
  Data : Inport
  Bus Selector : BusSelector  OutputSignals=SpeedRef,Speedfb,Id_Ref,Id_fb,Iq_Ref,Iq_fb,Ia,Ib,Pos_pu
  Data Store Read : DataStoreRead  DataStoreName=Debug_signals  IndexOptions=Index vector (dialog)  Indices=1  OutputSizes=1
  Demux : Demux  Outputs=2
  Ia_Ib : Constant  Value=[7 8]  OutDataTypeStr=uint16  SampleTime=-1
  Id_control2 : Constant  Value=[3 4]  OutDataTypeStr=uint16  SampleTime=-1
  Iq_control : Constant  Value=[5 6]  OutDataTypeStr=uint16  SampleTime=-1
  Multiport Switch : MultiPortSwitch  Inputs=4  DiagnosticForDefault=Warning  OutDataTypeStr=uint16  RndMeth=Simplest  SaturateOnIntegerOverflow=off  InputSameDT=off
  Mux : Mux  Inputs=8
  Selector : Selector  InputPortWidth=8  IndexOptions=Index vector (port)  Indices=[1 3]  OutputSizes=1
  Terminator : Terminator
  speed_control : Constant  Value=[1 2]  OutDataTypeStr=uint16  SampleTime=-1
  Debug_signal_1 : Outport
  Debug_signal_2 : Outport  Port=2
  wires:
  Demux/2 -> Debug_signal_2/1
  speed_control/1 -> Multiport Switch/2
  Selector/1 -> Demux/1
  Demux/1 -> Debug_signal_1/1
  Id_control2/1 -> Multiport Switch/3
  Iq_control/1 -> Multiport Switch/4
  Ia_Ib/1 -> Multiport Switch/5
  Multiport Switch/1 -> Selector/2
  Data Store Read/1 -> Multiport Switch/1
  Data/1 -> Bus Selector/1
  Bus Selector/2 -> Mux/2  "<Speedfb>"
  Mux/1 -> Selector/1
  Bus Selector/3 -> Mux/3  "<Id_Ref>"
  Bus Selector/4 -> Mux/4  "<Id_fb>"
  Bus Selector/5 -> Mux/5  "<Iq_Ref>"
  Bus Selector/6 -> Mux/6  "<Iq_fb>"
  Bus Selector/7 -> Mux/7  "<Ia>"
  Bus Selector/8 -> Mux/8  "<Ib>"
  Bus Selector/1 -> Mux/1  "<SpeedRef>"
  Bus Selector/9 -> Terminator/1  "<Pos_pu>"

== system foc_sensorless_am13x/Current loop/Initialize Driver and PWM Clock ==
  C Function : CFunction  CodeGenUsesSimCustomCode=off  CodegenInitializeConditionsCode=|  CodegenTerminateCode=DL_MCPWM_disableTBCLK();  CustomHeaderFile=|
      CodegenInitializeConditionsCode=|
      | /* Power-up adc converter core */
      | DL_ADC_powerUp(ADC_0_INST);
      | DL_ADC_powerUp(ADC_1_INST);
      | DL_ADC_powerUp(ADC_2_INST);
      | DEVICE_DELAY_US(10000); /* 10ms delay*/
      | /* Power-up MCPWM */
      | DL_MCPWM_enableTBCLK();
      | /* uart init */
      | mw_am13x_serial_Init();
      CustomHeaderFile=|
      | dl_gpio.h
      | hw_memmap.h
      | ti_sdk_dl_config.h
      | dl_mcpwm.h
      | dl_adc.h
  Constant1 : Constant  OutDataTypeStr=single
  Event Listener : EventListener  DisableCoverage=on  EventName=reset
  wires:
  Constant1/1 -> C Function/1

== system foc_sensorless_am13x/Current loop/Model Source ==

== system foc_sensorless_am13x/Current loop/Scale for AM13x PWM ==
  note: This gain is to create global variable for these signals, Its a workaround
  In1 : Inport
  Demux : Demux  Outputs=3
  Gain : Gain  OutDataTypeStr=uint16
  Gain1 : Gain  OutDataTypeStr=uint16
  Gain2 : Gain  OutDataTypeStr=uint16
  Scale_to_PWM_Counter_PRD : Gain  Gain=target.PWM_Counter_Period  OutDataTypeStr=uint16  RndMeth=Simplest
  Ua : Outport
  Ub : Outport  Port=2
  Uc : Outport  Port=3
  wires:
  Demux/2 -> Gain1/1
  Gain/1 -> Ua/1  "Ua"
  Demux/3 -> Gain2/1
  Gain2/1 -> Uc/1  "Uc"
  In1/1 -> Scale_to_PWM_Counter_PRD/1
  Demux/1 -> Gain/1
  Scale_to_PWM_Counter_PRD/1 -> Demux/1
  Gain1/1 -> Ub/1  "Ub"

== system foc_sensorless_am13x/Current loop/Serial Send ==
  SCI_Data : Inport
  Demux2 : Demux  Outputs=2
  While Iterator Subsystem : Subsystem  TreatAsAtomicUnit=on
  wires:
  Demux2/2 -> While Iterator Subsystem/2(Iteration)  "SCI_Tx_Iteration"
  Demux2/1 -> While Iterator Subsystem/1(Data)  "SCI_Tx_Data"
  SCI_Data/1 -> Demux2/1

== system foc_sensorless_am13x/Current loop/System Initialize ==

== system foc_sensorless_am13x/Current loop/System Outputs ==

== system foc_sensorless_am13x/Motor and Inverter/Get_PU ==
  In1 : Inport
  Constant : Constant  Value=2*pi  OutDataTypeStr=single
  Gain2 : Gain  Gain=1/(2*pi)  RndMeth=Simplest  OutDataTypeStr=Inherit: Same as input
  Mod : Math  Operator=mod
  Out1 : Outport
  wires:
  Constant/1 -> Mod/2
  In1/1 -> Mod/1
  Mod/1 -> Gain2/1
  Gain2/1 -> Out1/1

== system foc_sensorless_am13x/Motor and Inverter/Inverter ==
  Duty_abc : Inport
  Average-Value Inverter : mcbplantlib/Average-Value Inverter
  Constant2 : Constant  Value=inverter.V_dc  OutDataTypeStr=single  SampleTime=-1
  Data Type Conversion1 : DataTypeConversion  OutDataTypeStr=single  RndMeth=Simplest  SaturateOnIntegerOverflow=off
  Rate Transition3 : RateTransition  Deterministic=off  OutPortSampleTime=Ts_motor
  Vabc : Outport  VectorParamsAs1DForOutWhenUnconnected=off
  wires:
  Average-Value Inverter/1 -> Vabc/1
  Rate Transition3/1 -> Average-Value Inverter/1
  Duty_abc/1 -> Data Type Conversion1/1
  Data Type Conversion1/1 -> Rate Transition3/1
  Constant2/1 -> Average-Value Inverter/2

== system foc_sensorless_am13x/Motor and Inverter/Load_Profile (Torque) ==
  Constant : Constant  Value=.01*pmsm.T_rated  OutDataTypeStr=single  SampleTime=-1
  Data Type Conversion : DataTypeConversion  OutDataTypeStr=single  SaturateOnIntegerOverflow=off  RndMeth=Floor
  IIR Filter : mcbcontrolslib/IIR Filter  VariantControl=Low Pass Filter  VariantSelect=Low-pass  FilterConstantInputType=Specify via dialog  Filter_constant=0.001  InitialOutput=Specify via dialog  InitialOutputValue=0  ExternalReset=none  advancedSettings=off  Ts=50e-6  cutOff_freq=3.1863
  T_load : Step  Time=8  Before=.01*pmsm.T_rated  After=.05*pmsm.T_rated  SampleTime=Ts_motor
  Load_Trq : Outport  VectorParamsAs1DForOutWhenUnconnected=off
  wires:
  IIR Filter/1 -> Load_Trq/1
  Data Type Conversion/1 -> IIR Filter/1
  Constant/1 -> Data Type Conversion/1

== system foc_sensorless_am13x/Serial Receive/Model Header ==

== system foc_sensorless_am13x/Serial Receive/unParse ==
  Data : Inport
  Bitwise Operator : simulink/Logic and Bit Operations/Bitwise Operator  logicop=AND  UseBitMask=on  BitMask=hex2dec('0001')  BitMaskRealWorld=Stored Integer
  Bitwise Operator1 : simulink/Logic and Bit Operations/Bitwise Operator  logicop=AND  UseBitMask=on  BitMask=hex2dec('00F0')  BitMaskRealWorld=Stored Integer
  Data Type Conversion3 : DataTypeConversion  OutDataTypeStr=boolean  RndMeth=Simplest  SaturateOnIntegerOverflow=off
  Data Type Conversion4 : DataTypeConversion  OutDataTypeStr=uint16  RndMeth=Simplest  SaturateOnIntegerOverflow=off
  Shift Arithmetic1 : ArithShift  BitShiftNumber=4
  Enable_ClosedLoop : Outport
  Debug_signals : Outport  Port=2
  wires:
  Data Type Conversion3/1 -> Enable_ClosedLoop/1
  Shift Arithmetic1/1 -> Data Type Conversion4/1
  Data Type Conversion4/1 -> Debug_signals/1
  Bitwise Operator/1 -> Data Type Conversion3/1
  Data/1 -> Bitwise Operator1/1, Bitwise Operator/1
  Bitwise Operator1/1 -> Shift Arithmetic1/1

== system foc_sensorless_am13x/Speed loop/Iq_InitValue ==
  iq_latch : Inport
  wErr : Inport  Port=2
  Add : Sum  Inputs=-+  RndMeth=Simplest  OutDataTypeStr=Inherit: Same as first input
  Kp2 : Constant  Value=PI_params.Kp_speed  OutDataTypeStr=dataType  SampleTime=-1
  Product : Product  RndMeth=Simplest  OutDataTypeStr=Inherit: Same as first input
  Out1 : Outport
  wires:
  wErr/1 -> Product/2
  Add/1 -> Out1/1
  Product/1 -> Add/1
  Kp2/1 -> Product/1
  iq_latch/1 -> Add/2

== system foc_sensorless_am13x/Speed loop/System Outputs ==

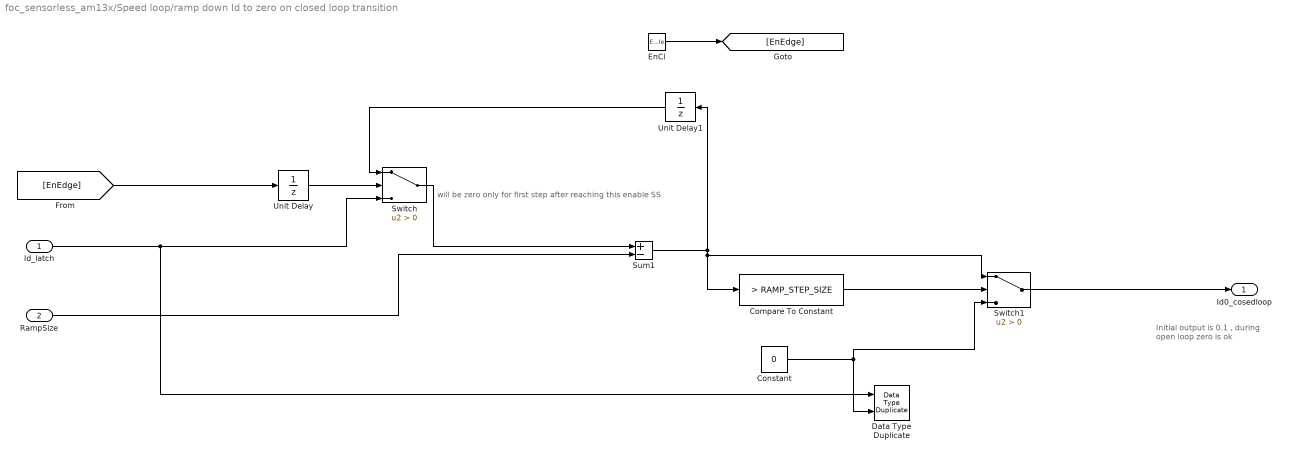
== system foc_sensorless_am13x/Speed loop/ramp down Id to zero on closed loop transition ==
  note: will be zero only for first step after reaching this enable SS
  note: Initial output is 0.1
      | , during open loop zero is ok
  Id_latch : Inport
  RampSize : Inport  Port=2
  EnCl : EnablePort  StatesWhenEnabling=reset  ShowOutputPort=on
  Compare To Constant : simulink/Logic and Bit Operations/Compare To Constant  relop=>  const=RAMP_STEP_SIZE  OutDataTypeStr=boolean
  Constant : Constant  Value=0  OutDataTypeStr=Inherit: Inherit via back propagation
  Data Type Duplicate : DataTypeDuplicate
  Sum1 : Sum  Inputs=+-  RndMeth=Simplest  OutDataTypeStr=Inherit: Same as first input
  Switch : Switch  Criteria=u2 > Threshold  SaturateOnIntegerOverflow=off  InputSameDT=off
  Switch1 : Switch  Criteria=u2 > Threshold  SaturateOnIntegerOverflow=off  InputSameDT=off
  Unit Delay : UnitDelay  SampleTime=-1  HasFrameUpgradeWarning=on
  Unit Delay1 : UnitDelay  SampleTime=-1  HasFrameUpgradeWarning=on
  Id0_cosedloop : Outport  InitialOutput=0
  wires:
  Id_latch/1 -> Switch/3, Data Type Duplicate/1
  Constant/1 -> Data Type Duplicate/2, Switch1/3
  Compare To Constant/1 -> Switch1/2
  Sum1/1 -> Unit Delay1/1, Compare To Constant/1, Switch1/1
  RampSize/1 -> Sum1/2
  Switch1/1 -> Id0_cosedloop/1
  EnCl/1 -> [EnEdge]
  [EnEdge] -> Unit Delay/1
  Unit Delay/1 -> Switch/2
  Unit Delay1/1 -> Switch/1
  Switch/1 -> Sum1/1

== system foc_sensorless_am13x/Current loop/Closed /Calculate Idq0 ==
  IdqRef : Inport
  IdqFb : Inport  Port=2
  Vdq0 : Inport  Port=3
  Add : Sum  Inputs=+-  RndMeth=Simplest  OutDataTypeStr=Inherit: Same as first input
  Add1 : Sum  Inputs=+-  RndMeth=Simplest  OutDataTypeStr=Inherit: Same as first input
  Kp : Constant  Value=PI_params.Kp_id  OutDataTypeStr=dataType  SampleTime=-1
  Product : Product  RndMeth=Simplest  OutDataTypeStr=Inherit: Same as first input
  Idq0 : Outport
  wires:
  IdqRef/1 -> Add1/1
  Add1/1 -> Product/1
  IdqFb/1 -> Add1/2
  Product/1 -> Add/2
  Vdq0/1 -> Add/1
  Kp/1 -> Product/2
  Add/1 -> Idq0/1

== system foc_sensorless_am13x/Current loop/Closed /Calculate VI Alpha Beta ==
  VICL : Inport
  EnCl : Inport  Port=2
  VOpen : Inport  Port=3
  Demux : Demux
  Switch : Switch  Criteria=u2 > Threshold  SaturateOnIntegerOverflow=off  InputSameDT=off
  Vector Concatenate : Concatenate
  Vector Concatenate1 : Concatenate
  Vector Concatenate2 : Concatenate
  VIAlphaBeta : Outport
  wires:
  VICL/1 -> Demux/1
  Demux/2 -> Vector Concatenate/2
  Demux/1 -> Vector Concatenate/1
  EnCl/1 -> Switch/2
  Vector Concatenate/1 -> Switch/1
  VOpen/1 -> Switch/3
  Vector Concatenate1/1 -> VIAlphaBeta/1
  Switch/1 -> Vector Concatenate1/1
  Demux/3 -> Vector Concatenate2/1
  Demux/4 -> Vector Concatenate2/2
  Vector Concatenate2/1 -> Vector Concatenate1/2

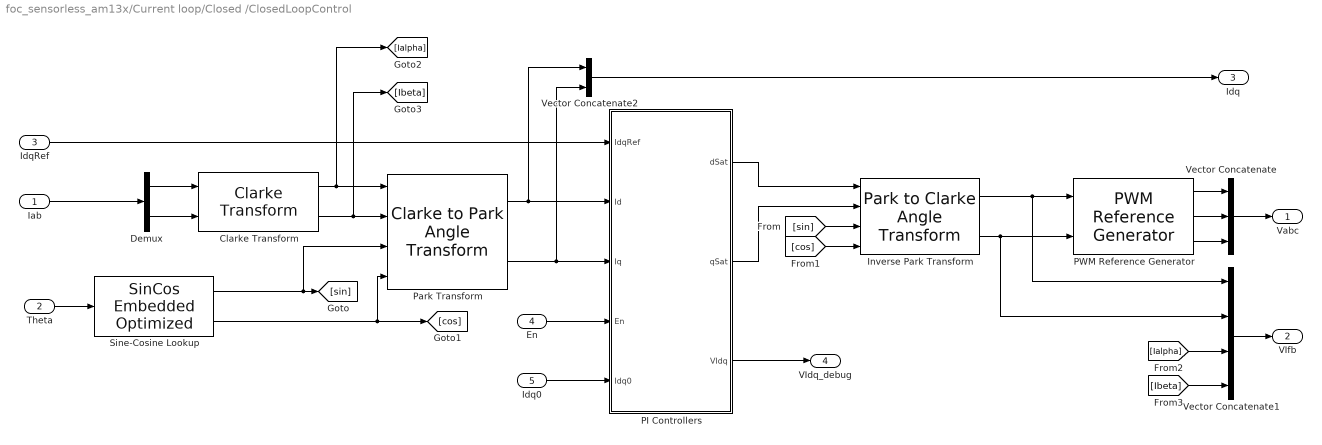
== system foc_sensorless_am13x/Current loop/Closed /ClosedLoopControl ==
  Iab : Inport
  Theta : Inport  Port=2
  IdqRef : Inport  Port=3
  En : Inport  Port=4
  Idq0 : Inport  Port=5
  Clarke Transform : mcbeeMathTransformLib/Clarke Transform  VariantControl=Variant2  PowerInvariant=off  UseWithEmbedded=on  PhaseInput=Two inputs
      settings: LibrarySourceBlock=mcblib/Controls/Math Transforms/Clarke Transform
  Demux : Demux  Outputs=2
  Inverse Park Transform : mcbeeMathTransformLib/Park to Clarke Angle Transform  AxisAlignment=D-axis  UseWithEmbedded=on  PhaseInput=Two inputs  ThetaInput=Sine and Cosine electrical position  AngleInput=Per-unit  N_points=1024
      settings: LibrarySourceBlock=mcblib/Controls/Math Transforms/Inverse Park Transform
  PI Controllers : Subsystem
  PWM Reference Generator : mcbcontrolslib/PWM Reference Generator  inSignal=Valphabeta  modType=SVM: space vector modulation
      settings: LibrarySourceBlock=mcblib/Controls/Math Transforms/PWM Reference Generator
  Park Transform : mcbeeMathTransformLib/Clarke to Park Angle Transform  AxisAlignment=D-axis  UseWithEmbedded=on  PhaseInput=Two inputs  ThetaInput=Sine and Cosine electrical position  AngleInput=Per-unit  N_points=1024
      settings: LibrarySourceBlock=mcblib/Controls/Math Transforms/Park Transform
  Sine-Cosine Lookup : mcbcontrolslib/SinCos Embedded Optimized  LabelModeActiveChoice=MCB_Sin  OptforProc=off  ApproximationMethod=None  UserApproxMethod=Lookup  ApproxStatus=None  InterpMethod=Linear point-slope  NumberOfDataPoints=16  NumberOfIterations=11  RemoveProtectionAgainstOutOfRangeInput=off  TableDataTypeStr=Inherit: Inherit via input  AngleInput=Per-unit  ThetaDataType=single  N_points=1024  DatatypeInput=Inherit from input  Datatype=Inherit: Same as input
      settings: LibrarySourceBlock=mcblib/Controls/Math Transforms/Sine-Cosine Lookup
  Vector Concatenate : Concatenate  NumInputs=3
  Vector Concatenate1 : Concatenate  NumInputs=4
  Vector Concatenate2 : Concatenate
  Vabc : Outport
  VIfb : Outport  Port=2
  Idq : Outport  Port=3
  VIdq_debug : Outport  Port=4  VectorParamsAs1DForOutWhenUnconnected=off
  wires:
  Demux/1 -> Clarke Transform/1
  Demux/2 -> Clarke Transform/2
  Clarke Transform/1 -> [Ialpha], Park Transform/1
  Clarke Transform/2 -> [Ibeta], Park Transform/2
  Sine-Cosine Lookup/1 -> [sin], Park Transform/3
  Sine-Cosine Lookup/2 -> Park Transform/4, [cos]
  Iab/1 -> Demux/1
  Theta/1 -> Sine-Cosine Lookup/1
  Inverse Park Transform/1 -> PWM Reference Generator/1, Vector Concatenate1/1
  Inverse Park Transform/2 -> PWM Reference Generator/2, Vector Concatenate1/2
  PWM Reference Generator/1 -> Vector Concatenate/1
  PWM Reference Generator/2 -> Vector Concatenate/2
  PWM Reference Generator/3 -> Vector Concatenate/3
  Vector Concatenate/1 -> Vabc/1
  Vector Concatenate1/1 -> VIfb/1
  IdqRef/1 -> PI Controllers/1(IdqRef)
  Park Transform/1 -> Vector Concatenate2/1, PI Controllers/2(Id)
  Park Transform/2 -> Vector Concatenate2/2, PI Controllers/3(Iq)
  En/1 -> PI Controllers/4(En)
  Idq0/1 -> PI Controllers/5(Idq0)
  Vector Concatenate2/1 -> Idq/1
  PI Controllers/1(dSat) -> Inverse Park Transform/1
  PI Controllers/2(qSat) -> Inverse Park Transform/2
  [sin] -> Inverse Park Transform/3
  [cos] -> Inverse Park Transform/4
  [Ialpha] -> Vector Concatenate1/3
  [Ibeta] -> Vector Concatenate1/4
  PI Controllers/3(VIdq) -> VIdq_debug/1

== system foc_sensorless_am13x/Current loop/Closed /Compensate ADC offset ==
  Iab_ADC : Inport
  Mode : Inport  Port=2
  Add : Sum  Inputs=-+  OutDataTypeStr=int16  RndMeth=Simplest
  Enabled Subsystem : Subsystem  TreatAsAtomicUnit=on
  Iab_ADC1 : InportShadow
  Invertering logic : Gain  Gain=inverter.invertingAmp  OutDataTypeStr=dataType
  NOT : Logic  Operator=NOT  IconShape=distinctive  AllPortsSameDT=off  OutDataTypeStr=boolean
  Scale to PU : Gain  Gain=1/2048  OutDataTypeStr=dataType
  Variant Source : VariantSource  VariantControlMode=sim codegen switching  ShowConditionOnBlock=on  VariantControls={(codegen), (sim)}
  ~1.65V in ADC counts : Constant  Value=[inverter.CtSensAOffset inverter.CtSensBOffset]  OutDataTypeStr=uint16  SampleTime=-1
  Iab_PU : Outport
  Iab_Offset : Outport  Port=2
  wires:
  Variant Source/1 -> Add/1
  Invertering logic/1 -> Iab_PU/1
  ~1.65V in ADC counts/1 -> Variant Source/2
  Enabled Subsystem/1(Iab_Offset) -> Iab_Offset/1, Variant Source/1
  Iab_ADC1/1 -> Enabled Subsystem/1(Iab_ADC)
  NOT/1 -> Enabled Subsystem/Enable
  Mode/1 -> NOT/1
  Scale to PU/1 -> Invertering logic/1
  Add/1 -> Scale to PU/1
  Iab_ADC/1 -> Add/2
